simulink model "ADLK"  (R2022a)
settings: Solver=FixedStepDiscrete  StartTime=0.0  StopTime=10.0  FixedStep=0.01  RelTol=1e-3
libraries: DoorRatSts x4, ADLKDriver x2
settings Model: Creator=DELL  LastModifiedBy=DELL
settings DataIOCC: SaveFormat=StructureWithTime
settings OptimizationCC: DefaultParameterBehavior=Inlined  EnhancedBackFolding=on  PassReuseOutputArgsAs=Individual arguments  ZeroExternalMemoryAtStartup=off  ZeroInternalMemoryAtStartup=off  OptimizeBlockOrder=speed  DifferentSizesBufferReuse=on  OptimizationCustomize=off  EfficientTunableParamExpr=on
settings DebuggingCC: ParameterTunabilityLossMsg=error
settings ModelReferenceCC: ModelReferenceNumInstancesAllowed=Single
settings SFSimCC: MATLABDynamicMemAlloc=off
settings RTWCC: Description=AUTOSAR  SystemTargetFile=autosar.tlc  GenCodeOnly=on  TemplateMakefile=ert_default_tmf
settings CodeAppCC: ForceParamTrailComments=on  IgnoreCustomStorageClasses=off  OperatorAnnotations=on  SimulinkDataObjDesc=on  SFDataObjDesc=on  InsertBlockDesc=on
settings STFCustomTargetCC: TargetLangStandard=C99 (ISO)  MultiwordLength=256  ParMdlRefBuildCompliant=on  CompOptLevelCompliant=on  IncludeMdlTerminateFcn=off  CombineOutputUpdateFcns=on  SuppressErrorStatus=on  ERTCustomFileBanners=on  SupportNonFinite=off  SupportComplex=off  SupportContinuousTime=off  SupportNonInlinedSFcns=off  RemoveResetFunc=on  MATLABClassNameForMDSCustomization=Simulink.SoftwareTarget.ERTCustomization  AutosarCompliant=on  GRTInterface=off  UseToolchainInfoCompliant=on  LookupTableObjectStructAxisOrder=2,1,3,4,...  LUTObjectStructOrderEvenSpacing=Size,Table,Breakpoints  SystemTargetFile=autosar.tlc
settings ERTTargetCC: TargetLangStandard=C99 (ISO)  ConcurrentExecutionCompliant=off  IncludeMdlTerminateFcn=off  SuppressErrorStatus=on  SupportNonFinite=off  SupportComplex=off  ModelStepFunctionPrototypeControlCompliant=off  CPPClassGenCompliant=off  AutosarCompliant=on  LookupTableObjectStructAxisOrder=2,1,3,4,...  LUTObjectStructOrderEvenSpacing=Size,Table,Breakpoints  InlinedParameterPlacement=NonHierarchical  ERTCustomFileTemplate=example_file_process.tlc

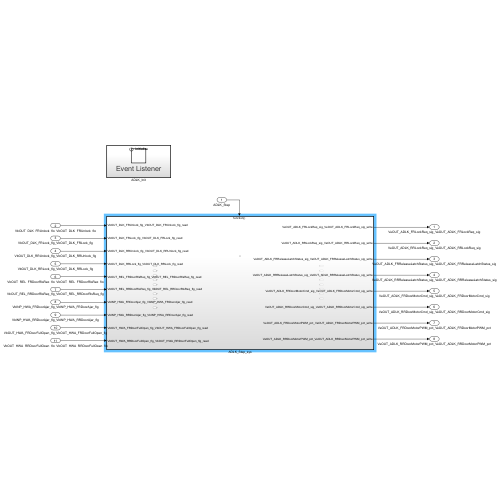
[thumbnail: Simulink's stored preview of the top-level diagram]
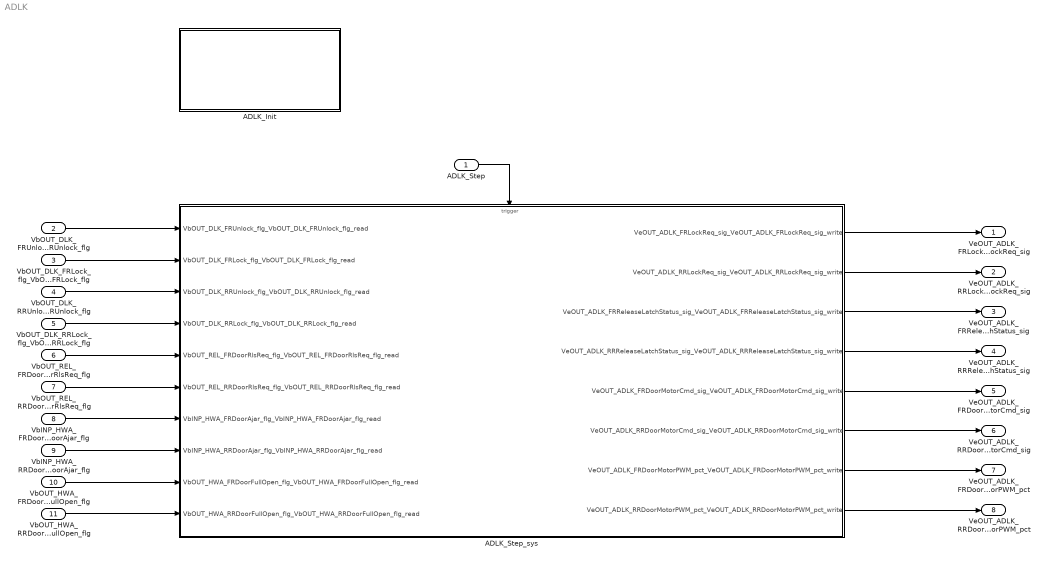
== system ADLK ==
  ADLK_Step : Inport  SampleTime=0.01  OutputFunctionCall=on
  VbOUT_DLK_FRUnlock_flg_VbOUT_DLK_FRUnlock_flg : Inport  Port=2  OutDataTypeStr=Boolean  PortDimensions=1
  VbOUT_DLK_FRLock_flg_VbOUT_DLK_FRLock_flg : Inport  Port=3  OutDataTypeStr=Boolean  PortDimensions=1
  VbOUT_DLK_RRUnlock_flg_VbOUT_DLK_RRUnlock_flg : Inport  Port=4  OutDataTypeStr=Boolean  PortDimensions=1
  VbOUT_DLK_RRLock_flg_VbOUT_DLK_RRLock_flg : Inport  Port=5  OutDataTypeStr=Boolean  PortDimensions=1
  VbOUT_REL_FRDoorRlsReq_flg_VbOUT_REL_FRDoorRlsReq_flg : Inport  Port=6  OutDataTypeStr=Boolean  PortDimensions=1
  VbOUT_REL_RRDoorRlsReq_flg_VbOUT_REL_RRDoorRlsReq_flg : Inport  Port=7  OutDataTypeStr=Boolean  PortDimensions=1
  VbINP_HWA_FRDoorAjar_flg_VbINP_HWA_FRDoorAjar_flg : Inport  Port=8  OutDataTypeStr=Boolean  PortDimensions=1
  VbINP_HWA_RRDoorAjar_flg_VbINP_HWA_RRDoorAjar_flg : Inport  Port=9  OutDataTypeStr=Boolean  PortDimensions=1
  VbOUT_HWA_FRDoorFullOpen_flg_VbOUT_HWA_FRDoorFullOpen_flg : Inport  Port=10  OutDataTypeStr=Boolean  PortDimensions=1
  VbOUT_HWA_RRDoorFullOpen_flg_VbOUT_HWA_RRDoorFullOpen_flg : Inport  Port=11  OutDataTypeStr=Boolean  PortDimensions=1
  ADLK_Init : Subsystem
  ADLK_Step_sys : Subsystem
  VeOUT_ADLK_FRLockReq_sig_VeOUT_ADLK_FRLockReq_sig : Outport  OutDataTypeStr=UInt8  PortDimensions=1
  VeOUT_ADLK_RRLockReq_sig_VeOUT_ADLK_RRLockReq_sig : Outport  Port=2  OutDataTypeStr=UInt8  PortDimensions=1
  VeOUT_ADLK_FRReleaseLatchStatus_sig_VeOUT_ADLK_FRReleaseLatchStatus_sig : Outport  Port=3  OutDataTypeStr=UInt8  PortDimensions=1
  VeOUT_ADLK_RRReleaseLatchStatus_sig_VeOUT_ADLK_RRReleaseLatchStatus_sig : Outport  Port=4  OutDataTypeStr=UInt8  PortDimensions=1
  VeOUT_ADLK_FRDoorMotorCmd_sig_VeOUT_ADLK_FRDoorMotorCmd_sig : Outport  Port=5  OutDataTypeStr=UInt8  PortDimensions=1
  VeOUT_ADLK_RRDoorMotorCmd_sig_VeOUT_ADLK_RRDoorMotorCmd_sig : Outport  Port=6  OutDataTypeStr=UInt8  PortDimensions=1
  VeOUT_ADLK_FRDoorMotorPWM_pct_VeOUT_ADLK_FRDoorMotorPWM_pct : Outport  Port=7  OutDataTypeStr=UInt8  PortDimensions=1
  VeOUT_ADLK_RRDoorMotorPWM_pct_VeOUT_ADLK_RRDoorMotorPWM_pct : Outport  Port=8  OutDataTypeStr=UInt8  PortDimensions=1
  wires:
  VbOUT_DLK_FRUnlock_flg_VbOUT_DLK_FRUnlock_flg/1 -> ADLK_Step_sys/1(VbOUT_DLK_FRUnlock_flg_VbOUT_DLK_FRUnlock_flg_read)
  VbOUT_DLK_FRLock_flg_VbOUT_DLK_FRLock_flg/1 -> ADLK_Step_sys/2(VbOUT_DLK_FRLock_flg_VbOUT_DLK_FRLock_flg_read)
  VbOUT_DLK_RRUnlock_flg_VbOUT_DLK_RRUnlock_flg/1 -> ADLK_Step_sys/3(VbOUT_DLK_RRUnlock_flg_VbOUT_DLK_RRUnlock_flg_read)
  VbOUT_DLK_RRLock_flg_VbOUT_DLK_RRLock_flg/1 -> ADLK_Step_sys/4(VbOUT_DLK_RRLock_flg_VbOUT_DLK_RRLock_flg_read)
  VbOUT_REL_FRDoorRlsReq_flg_VbOUT_REL_FRDoorRlsReq_flg/1 -> ADLK_Step_sys/5(VbOUT_REL_FRDoorRlsReq_flg_VbOUT_REL_FRDoorRlsReq_flg_read)
  VbOUT_REL_RRDoorRlsReq_flg_VbOUT_REL_RRDoorRlsReq_flg/1 -> ADLK_Step_sys/6(VbOUT_REL_RRDoorRlsReq_flg_VbOUT_REL_RRDoorRlsReq_flg_read)
  VbINP_HWA_FRDoorAjar_flg_VbINP_HWA_FRDoorAjar_flg/1 -> ADLK_Step_sys/7(VbINP_HWA_FRDoorAjar_flg_VbINP_HWA_FRDoorAjar_flg_read)
  VbINP_HWA_RRDoorAjar_flg_VbINP_HWA_RRDoorAjar_flg/1 -> ADLK_Step_sys/8(VbINP_HWA_RRDoorAjar_flg_VbINP_HWA_RRDoorAjar_flg_read)
  VbOUT_HWA_FRDoorFullOpen_flg_VbOUT_HWA_FRDoorFullOpen_flg/1 -> ADLK_Step_sys/9(VbOUT_HWA_FRDoorFullOpen_flg_VbOUT_HWA_FRDoorFullOpen_flg_read)
  VbOUT_HWA_RRDoorFullOpen_flg_VbOUT_HWA_RRDoorFullOpen_flg/1 -> ADLK_Step_sys/10(VbOUT_HWA_RRDoorFullOpen_flg_VbOUT_HWA_RRDoorFullOpen_flg_read)
  ADLK_Step_sys/1(VeOUT_ADLK_FRLockReq_sig_VeOUT_ADLK_FRLockReq_sig_write) -> VeOUT_ADLK_FRLockReq_sig_VeOUT_ADLK_FRLockReq_sig/1
  ADLK_Step_sys/2(VeOUT_ADLK_RRLockReq_sig_VeOUT_ADLK_RRLockReq_sig_write) -> VeOUT_ADLK_RRLockReq_sig_VeOUT_ADLK_RRLockReq_sig/1
  ADLK_Step_sys/3(VeOUT_ADLK_FRReleaseLatchStatus_sig_VeOUT_ADLK_FRReleaseLatchStatus_sig_write) -> VeOUT_ADLK_FRReleaseLatchStatus_sig_VeOUT_ADLK_FRReleaseLatchStatus_sig/1
  ADLK_Step_sys/4(VeOUT_ADLK_RRReleaseLatchStatus_sig_VeOUT_ADLK_RRReleaseLatchStatus_sig_write) -> VeOUT_ADLK_RRReleaseLatchStatus_sig_VeOUT_ADLK_RRReleaseLatchStatus_sig/1
  ADLK_Step_sys/5(VeOUT_ADLK_FRDoorMotorCmd_sig_VeOUT_ADLK_FRDoorMotorCmd_sig_write) -> VeOUT_ADLK_FRDoorMotorCmd_sig_VeOUT_ADLK_FRDoorMotorCmd_sig/1
  ADLK_Step_sys/6(VeOUT_ADLK_RRDoorMotorCmd_sig_VeOUT_ADLK_RRDoorMotorCmd_sig_write) -> VeOUT_ADLK_RRDoorMotorCmd_sig_VeOUT_ADLK_RRDoorMotorCmd_sig/1
  ADLK_Step_sys/7(VeOUT_ADLK_FRDoorMotorPWM_pct_VeOUT_ADLK_FRDoorMotorPWM_pct_write) -> VeOUT_ADLK_FRDoorMotorPWM_pct_VeOUT_ADLK_FRDoorMotorPWM_pct/1
  ADLK_Step_sys/8(VeOUT_ADLK_RRDoorMotorPWM_pct_VeOUT_ADLK_RRDoorMotorPWM_pct_write) -> VeOUT_ADLK_RRDoorMotorPWM_pct_VeOUT_ADLK_RRDoorMotorPWM_pct/1
  ADLK_Step/1 -> ADLK_Step_sys/Trigger

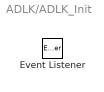
== system ADLK/ADLK_Init ==
  Event Listener : EventListener  EventName=reset

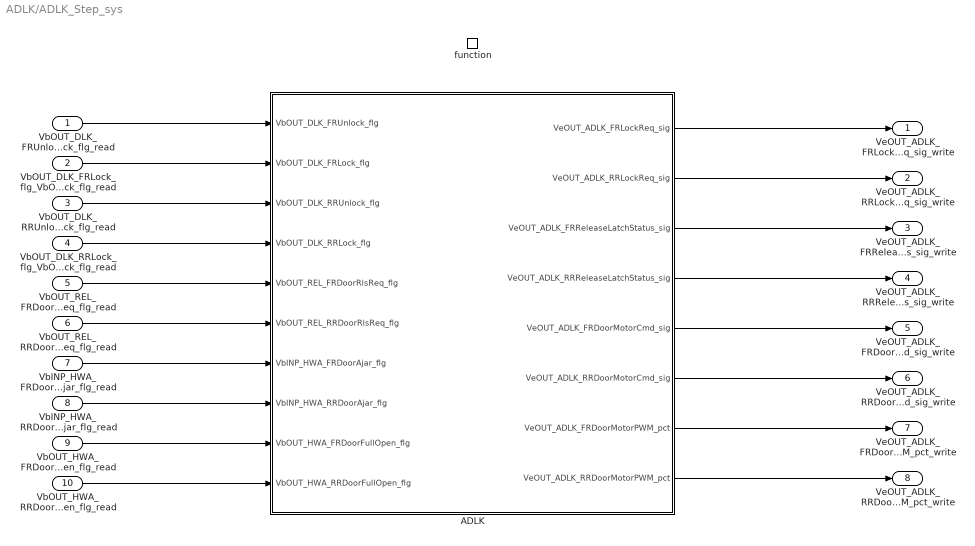
== system ADLK/ADLK_Step_sys ==
  VbOUT_DLK_FRUnlock_flg_VbOUT_DLK_FRUnlock_flg_read : Inport
  VbOUT_DLK_FRLock_flg_VbOUT_DLK_FRLock_flg_read : Inport  Port=2
  VbOUT_DLK_RRUnlock_flg_VbOUT_DLK_RRUnlock_flg_read : Inport  Port=3
  VbOUT_DLK_RRLock_flg_VbOUT_DLK_RRLock_flg_read : Inport  Port=4
  VbOUT_REL_FRDoorRlsReq_flg_VbOUT_REL_FRDoorRlsReq_flg_read : Inport  Port=5
  VbOUT_REL_RRDoorRlsReq_flg_VbOUT_REL_RRDoorRlsReq_flg_read : Inport  Port=6
  VbINP_HWA_FRDoorAjar_flg_VbINP_HWA_FRDoorAjar_flg_read : Inport  Port=7
  VbINP_HWA_RRDoorAjar_flg_VbINP_HWA_RRDoorAjar_flg_read : Inport  Port=8
  VbOUT_HWA_FRDoorFullOpen_flg_VbOUT_HWA_FRDoorFullOpen_flg_read : Inport  Port=9
  VbOUT_HWA_RRDoorFullOpen_flg_VbOUT_HWA_RRDoorFullOpen_flg_read : Inport  Port=10
  function : TriggerPort  TriggerType=function-call  VariantControl=(inherit)  SampleTimeType=periodic  SampleTime=-1
  ADLK : Subsystem
  VeOUT_ADLK_FRLockReq_sig_VeOUT_ADLK_FRLockReq_sig_write : Outport
      settings: EnsureOutportIsVirtual=on
  VeOUT_ADLK_RRLockReq_sig_VeOUT_ADLK_RRLockReq_sig_write : Outport  Port=2
      settings: EnsureOutportIsVirtual=on
  VeOUT_ADLK_FRReleaseLatchStatus_sig_VeOUT_ADLK_FRReleaseLatchStatus_sig_write : Outport  Port=3
      settings: EnsureOutportIsVirtual=on
  VeOUT_ADLK_RRReleaseLatchStatus_sig_VeOUT_ADLK_RRReleaseLatchStatus_sig_write : Outport  Port=4
      settings: EnsureOutportIsVirtual=on
  VeOUT_ADLK_FRDoorMotorCmd_sig_VeOUT_ADLK_FRDoorMotorCmd_sig_write : Outport  Port=5
      settings: EnsureOutportIsVirtual=on
  VeOUT_ADLK_RRDoorMotorCmd_sig_VeOUT_ADLK_RRDoorMotorCmd_sig_write : Outport  Port=6
      settings: EnsureOutportIsVirtual=on
  VeOUT_ADLK_FRDoorMotorPWM_pct_VeOUT_ADLK_FRDoorMotorPWM_pct_write : Outport  Port=7
      settings: EnsureOutportIsVirtual=on
  VeOUT_ADLK_RRDoorMotorPWM_pct_VeOUT_ADLK_RRDoorMotorPWM_pct_write : Outport  Port=8
      settings: EnsureOutportIsVirtual=on
  wires:
  VbOUT_DLK_FRUnlock_flg_VbOUT_DLK_FRUnlock_flg_read/1 -> ADLK/1(VbOUT_DLK_FRUnlock_flg)
  VbOUT_DLK_FRLock_flg_VbOUT_DLK_FRLock_flg_read/1 -> ADLK/2(VbOUT_DLK_FRLock_flg)
  VbOUT_DLK_RRUnlock_flg_VbOUT_DLK_RRUnlock_flg_read/1 -> ADLK/3(VbOUT_DLK_RRUnlock_flg)
  VbOUT_DLK_RRLock_flg_VbOUT_DLK_RRLock_flg_read/1 -> ADLK/4(VbOUT_DLK_RRLock_flg)
  VbOUT_REL_FRDoorRlsReq_flg_VbOUT_REL_FRDoorRlsReq_flg_read/1 -> ADLK/5(VbOUT_REL_FRDoorRlsReq_flg)
  VbOUT_REL_RRDoorRlsReq_flg_VbOUT_REL_RRDoorRlsReq_flg_read/1 -> ADLK/6(VbOUT_REL_RRDoorRlsReq_flg)
  VbINP_HWA_FRDoorAjar_flg_VbINP_HWA_FRDoorAjar_flg_read/1 -> ADLK/7(VbINP_HWA_FRDoorAjar_flg)
  VbINP_HWA_RRDoorAjar_flg_VbINP_HWA_RRDoorAjar_flg_read/1 -> ADLK/8(VbINP_HWA_RRDoorAjar_flg)
  VbOUT_HWA_FRDoorFullOpen_flg_VbOUT_HWA_FRDoorFullOpen_flg_read/1 -> ADLK/9(VbOUT_HWA_FRDoorFullOpen_flg)
  VbOUT_HWA_RRDoorFullOpen_flg_VbOUT_HWA_RRDoorFullOpen_flg_read/1 -> ADLK/10(VbOUT_HWA_RRDoorFullOpen_flg)
  ADLK/1(VeOUT_ADLK_FRLockReq_sig) -> VeOUT_ADLK_FRLockReq_sig_VeOUT_ADLK_FRLockReq_sig_write/1
  ADLK/2(VeOUT_ADLK_RRLockReq_sig) -> VeOUT_ADLK_RRLockReq_sig_VeOUT_ADLK_RRLockReq_sig_write/1
  ADLK/3(VeOUT_ADLK_FRReleaseLatchStatus_sig) -> VeOUT_ADLK_FRReleaseLatchStatus_sig_VeOUT_ADLK_FRReleaseLatchStatus_sig_write/1
  ADLK/4(VeOUT_ADLK_RRReleaseLatchStatus_sig) -> VeOUT_ADLK_RRReleaseLatchStatus_sig_VeOUT_ADLK_RRReleaseLatchStatus_sig_write/1
  ADLK/5(VeOUT_ADLK_FRDoorMotorCmd_sig) -> VeOUT_ADLK_FRDoorMotorCmd_sig_VeOUT_ADLK_FRDoorMotorCmd_sig_write/1
  ADLK/6(VeOUT_ADLK_RRDoorMotorCmd_sig) -> VeOUT_ADLK_RRDoorMotorCmd_sig_VeOUT_ADLK_RRDoorMotorCmd_sig_write/1
  ADLK/7(VeOUT_ADLK_FRDoorMotorPWM_pct) -> VeOUT_ADLK_FRDoorMotorPWM_pct_VeOUT_ADLK_FRDoorMotorPWM_pct_write/1
  ADLK/8(VeOUT_ADLK_RRDoorMotorPWM_pct) -> VeOUT_ADLK_RRDoorMotorPWM_pct_VeOUT_ADLK_RRDoorMotorPWM_pct_write/1

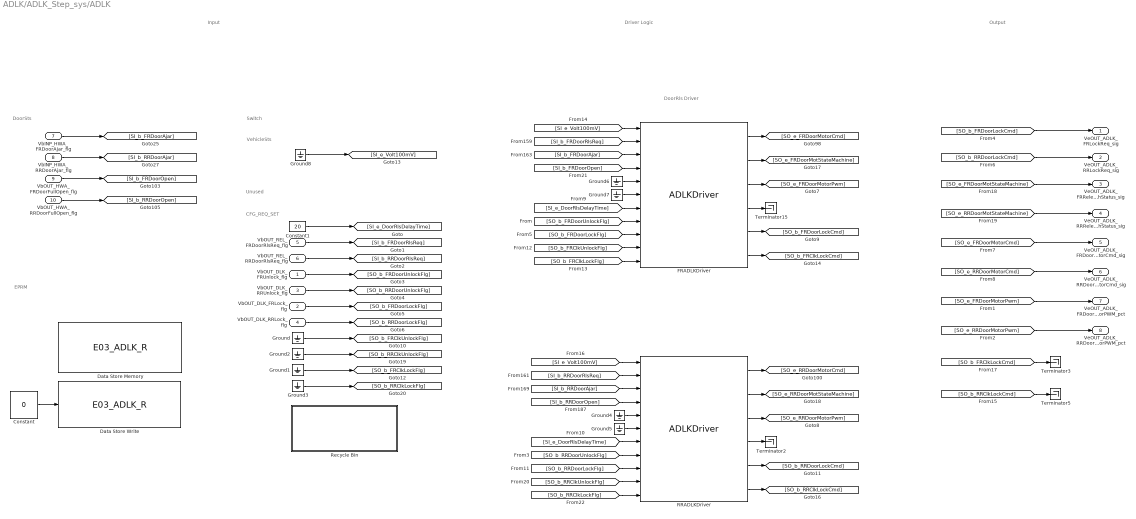
== system ADLK/ADLK_Step_sys/ADLK ==
  note: VehicleSts
  note: Input
  note: Output
  note: EPRM
  note: Driver Logic
  note: DoorRls Driver
  note: Switch
  note: DoorSts
  note: CFG_REQ_SET
  note: Unused
  VbOUT_DLK_FRUnlock_flg : Inport
  VbOUT_DLK_FRLock_flg : Inport  Port=2
  VbOUT_DLK_RRUnlock_flg : Inport  Port=3
  VbOUT_DLK_RRLock_flg : Inport  Port=4
  VbOUT_REL_FRDoorRlsReq_flg : Inport  Port=5
  VbOUT_REL_RRDoorRlsReq_flg : Inport  Port=6
  VbINP_HWA_FRDoorAjar_flg : Inport  Port=7
  VbINP_HWA_RRDoorAjar_flg : Inport  Port=8
  VbOUT_HWA_FRDoorFullOpen_flg : Inport  Port=9
  VbOUT_HWA_RRDoorFullOpen_flg : Inport  Port=10
  Constant : Constant  Value=0  OutDataTypeStr=uint8
  Constant1 : Constant  Value=20  OutDataTypeStr=uint8
  Data Store Memory : DataStoreMemory  DataStoreName=E03_ADLK_R  WriteAfterWriteMsg=warning  ShowAdditionalParam=off  OutDataTypeStr=uint8
  Data Store Write : DataStoreWrite  DataStoreName=E03_ADLK_R  IndexOptions=Index vector (dialog)  Indices=1  OutputSizes=1
  FRADLKDriver : ADLKDriver/ADLKDriver  SystemSampleTime=-1  VariantActivationTime=update diagram  Latency=0  AutoFrameSizeCalculation=off
  Ground{,1..8} (9 alike) : Ground
  RRADLKDriver : ADLKDriver/ADLKDriver  SystemSampleTime=-1  VariantActivationTime=update diagram  Latency=0  AutoFrameSizeCalculation=off
  Recycle Bin : Subsystem
  Terminator{2..3,5,15} (4 alike) : Terminator
  VeOUT_ADLK_FRLockReq_sig : Outport
  VeOUT_ADLK_RRLockReq_sig : Outport  Port=2
  VeOUT_ADLK_FRReleaseLatchStatus_sig : Outport  Port=3
  VeOUT_ADLK_RRReleaseLatchStatus_sig : Outport  Port=4
  VeOUT_ADLK_FRDoorMotorCmd_sig : Outport  Port=5
  VeOUT_ADLK_RRDoorMotorCmd_sig : Outport  Port=6
  VeOUT_ADLK_FRDoorMotorPWM_pct : Outport  Port=7
  VeOUT_ADLK_RRDoorMotorPWM_pct : Outport  Port=8
  wires:
  Constant/1 -> Data Store Write/1
  [SI_b_RRDoorOpen] -> RRADLKDriver/4
  [SI_b_RRDoorAjar] -> RRADLKDriver/3
  [SI_b_RRDoorRlsReq] -> RRADLKDriver/2
  [SI_e_Volt100mV] -> RRADLKDriver/1
  [SI_b_FRDoorAjar] -> FRADLKDriver/3
  [SI_b_FRDoorRlsReq] -> FRADLKDriver/2
  [SI_b_FRDoorOpen] -> FRADLKDriver/4
  [SI_e_DoorRlsDelayTime] -> FRADLKDriver/7
  Ground4/1 -> RRADLKDriver/5
  Ground5/1 -> RRADLKDriver/6
  Ground6/1 -> FRADLKDriver/5
  Ground7/1 -> FRADLKDriver/6
  [SI_e_Volt100mV] -> FRADLKDriver/1
  Constant1/1 -> [SI_e_DoorRlsDelayTime]
  [SI_e_DoorRlsDelayTime] -> RRADLKDriver/7
  [SO_b_FRDoorLockFlg] -> FRADLKDriver/9
  [SO_b_FRDoorUnlockFlg] -> FRADLKDriver/8
  [SO_b_RRDoorUnlockFlg] -> RRADLKDriver/8
  [SO_b_RRDoorLockFlg] -> RRADLKDriver/9
  [SO_b_FRClkUnlockFlg] -> FRADLKDriver/10
  [SO_b_FRClkLockFlg] -> FRADLKDriver/11
  Ground/1 -> [SO_b_FRClkUnlockFlg]
  Ground1/1 -> [SO_b_FRClkLockFlg]
  [SO_b_FRDoorLockCmd] -> VeOUT_ADLK_FRLockReq_sig/1
  [SO_b_RRDoorLockCmd] -> VeOUT_ADLK_RRLockReq_sig/1
  [SO_e_FRDoorMotStateMachine] -> VeOUT_ADLK_FRReleaseLatchStatus_sig/1
  [SO_e_RRDoorMotStateMachine] -> VeOUT_ADLK_RRReleaseLatchStatus_sig/1
  [SO_b_FRClkLockCmd] -> Terminator3/1
  [SO_b_RRClkLockCmd] -> Terminator5/1
  Ground2/1 -> [SO_b_RRClkUnlockFlg]
  Ground3/1 -> [SO_b_RRClkLockFlg]
  [SO_b_RRClkUnlockFlg] -> RRADLKDriver/10
  [SO_b_RRClkLockFlg] -> RRADLKDriver/11
  VbINP_HWA_FRDoorAjar_flg/1 -> [SI_b_FRDoorAjar]
  VbINP_HWA_RRDoorAjar_flg/1 -> [SI_b_RRDoorAjar]
  VbOUT_HWA_FRDoorFullOpen_flg/1 -> [SI_b_FRDoorOpen]
  VbOUT_HWA_RRDoorFullOpen_flg/1 -> [SI_b_RRDoorOpen]
  VbOUT_REL_FRDoorRlsReq_flg/1 -> [SI_b_FRDoorRlsReq]
  VbOUT_REL_RRDoorRlsReq_flg/1 -> [SI_b_RRDoorRlsReq]
  VbOUT_DLK_FRUnlock_flg/1 -> [SO_b_FRDoorUnlockFlg]
  VbOUT_DLK_RRUnlock_flg/1 -> [SO_b_RRDoorUnlockFlg]
  VbOUT_DLK_FRLock_flg/1 -> [SO_b_FRDoorLockFlg]
  VbOUT_DLK_RRLock_flg/1 -> [SO_b_RRDoorLockFlg]
  RRADLKDriver/3 -> [SO_e_RRDoorMotorPwm]
  [SO_e_FRDoorMotorCmd] -> VeOUT_ADLK_FRDoorMotorCmd_sig/1
  [SO_e_RRDoorMotorCmd] -> VeOUT_ADLK_RRDoorMotorCmd_sig/1
  [SO_e_FRDoorMotorPwm] -> VeOUT_ADLK_FRDoorMotorPWM_pct/1
  [SO_e_RRDoorMotorPwm] -> VeOUT_ADLK_RRDoorMotorPWM_pct/1
  FRADLKDriver/3 -> [SO_e_FRDoorMotorPwm]
  FRADLKDriver/1 -> [SO_e_FRDoorMotorCmd]
  FRADLKDriver/4 -> Terminator15/1
  FRADLKDriver/6 -> [SO_b_FRClkLockCmd]
  FRADLKDriver/5 -> [SO_b_FRDoorLockCmd]
  FRADLKDriver/2 -> [SO_e_FRDoorMotStateMachine]
  RRADLKDriver/1 -> [SO_e_RRDoorMotorCmd]
  RRADLKDriver/6 -> [SO_b_RRClkLockCmd]
  RRADLKDriver/5 -> [SO_b_RRDoorLockCmd]
  RRADLKDriver/2 -> [SO_e_RRDoorMotStateMachine]
  RRADLKDriver/4 -> Terminator2/1
  Ground8/1 -> [SI_e_Volt100mV]

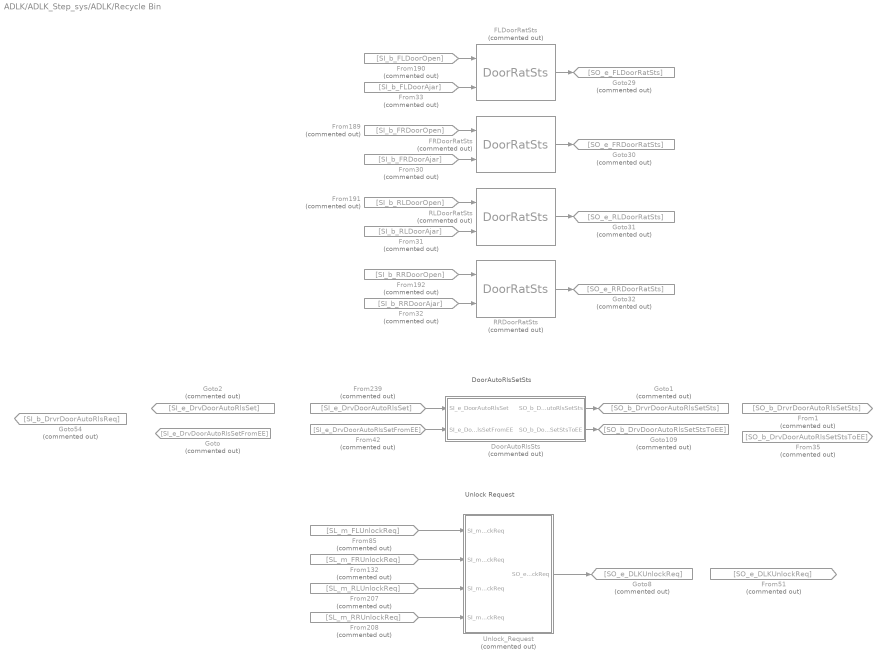
== system ADLK/ADLK_Step_sys/ADLK/Recycle Bin ==
  note: DoorAutoRlsSetSts
  note: Unlock Request
  DoorAutoRlsSts : Stateflow chart  Commented=on  TreatAsAtomicUnit=on
  FLDoorRatSts : DoorRatSts/DoorRatSts  Commented=on  SystemSampleTime=-1  VariantActivationTime=update diagram  Latency=0  AutoFrameSizeCalculation=off
  FRDoorRatSts : DoorRatSts/DoorRatSts  Commented=on  SystemSampleTime=-1  VariantActivationTime=update diagram  Latency=0  AutoFrameSizeCalculation=off
  From1 : From  Commented=on  GotoTag=SO_b_DrvrDoorAutoRlsSetSts
  From132 : From  Commented=on  GotoTag=SL_m_FRUnlockReq
  From189 : From  Commented=on  GotoTag=SI_b_FRDoorOpen
  From190 : From  Commented=on  GotoTag=SI_b_FLDoorOpen
  From191 : From  Commented=on  GotoTag=SI_b_RLDoorOpen
  From192 : From  Commented=on  GotoTag=SI_b_RRDoorOpen
  From207 : From  Commented=on  GotoTag=SL_m_RLUnlockReq
  From208 : From  Commented=on  GotoTag=SL_m_RRUnlockReq
  From239 : From  Commented=on  GotoTag=SI_e_DrvDoorAutoRlsSet
  From30 : From  Commented=on  GotoTag=SI_b_FRDoorAjar
  From31 : From  Commented=on  GotoTag=SI_b_RLDoorAjar
  From32 : From  Commented=on  GotoTag=SI_b_RRDoorAjar
  From33 : From  Commented=on  GotoTag=SI_b_FLDoorAjar
  From35 : From  Commented=on  GotoTag=SO_b_DrvDoorAutoRlsSetStsToEE
  From42 : From  Commented=on  GotoTag=SI_e_DrvDoorAutoRlsSetFromEE
  From51 : From  Commented=on  GotoTag=SO_e_DLKUnlockReq
  From85 : From  Commented=on  GotoTag=SL_m_FLUnlockReq
  Goto : Goto  Commented=on  GotoTag=SI_e_DrvDoorAutoRlsSetFromEE
  Goto1 : Goto  Commented=on  GotoTag=SO_b_DrvrDoorAutoRlsSetSts
  Goto109 : Goto  Commented=on  GotoTag=SO_b_DrvDoorAutoRlsSetStsToEE
  Goto2 : Goto  Commented=on  GotoTag=SI_e_DrvDoorAutoRlsSet
  Goto29 : Goto  Commented=on  GotoTag=SO_e_FLDoorRatSts
  Goto30 : Goto  Commented=on  GotoTag=SO_e_FRDoorRatSts
  Goto31 : Goto  Commented=on  GotoTag=SO_e_RLDoorRatSts
  Goto32 : Goto  Commented=on  GotoTag=SO_e_RRDoorRatSts
  Goto54 : Goto  Commented=on  GotoTag=SI_b_DrvrDoorAutoRlsReq
  Goto8 : Goto  Commented=on  GotoTag=SO_e_DLKUnlockReq
  RLDoorRatSts : DoorRatSts/DoorRatSts  Commented=on  SystemSampleTime=-1  VariantActivationTime=update diagram  Latency=0  AutoFrameSizeCalculation=off
  RRDoorRatSts : DoorRatSts/DoorRatSts  Commented=on  SystemSampleTime=-1  VariantActivationTime=update diagram  Latency=0  AutoFrameSizeCalculation=off
  Unlock_Request : Stateflow chart  Commented=on  TreatAsAtomicUnit=on
  wires:
  FLDoorRatSts/1 -> Goto29/1
  From191/1 -> RLDoorRatSts/1
  FRDoorRatSts/1 -> Goto30/1
  From190/1 -> FLDoorRatSts/1
  From192/1 -> RRDoorRatSts/1
  From189/1 -> FRDoorRatSts/1
  RRDoorRatSts/1 -> Goto32/1
  RLDoorRatSts/1 -> Goto31/1
  From30/1 -> FRDoorRatSts/2
  From32/1 -> RRDoorRatSts/2
  From31/1 -> RLDoorRatSts/2
  From33/1 -> FLDoorRatSts/2
  DoorAutoRlsSts/1(SO_b_DoorAutoRlsSetSts) -> Goto1/1
  DoorAutoRlsSts/2(SO_b_DoorAutoRlsSetStsToEE) -> Goto109/1
  From42/1 -> DoorAutoRlsSts/2(SI_e_DoorAutoRlsSetFromEE)
  From239/1 -> DoorAutoRlsSts/1(SI_e_DoorAutoRlsSet)
  From132/1 -> Unlock_Request/2(SI_m_FRUnlockReq)
  From208/1 -> Unlock_Request/4(SI_m_RRUnlockReq)
  From207/1 -> Unlock_Request/3(SI_m_RLUnlockReq)
  Unlock_Request/1(SO_e_UnlockReq) -> Goto8/1
  From85/1 -> Unlock_Request/1(SI_m_FLUnlockReq)

== stateflow chart ADLK/ADLK_Step_sys/ADLK/Recycle Bin/DoorAutoRlsSts ==
  state DoorLockSet
    (default) -> (junction 127) : /* DoorLockSet */
    DoorLockSet -> (junction 127)
    (junction 127) -> (junction 128) [order 1] : [SI_e_DoorAutoRlsSet == 1 || ...
        | (SI_e_DoorAutoRlsSet != 2 && SL_e_DoorAutoRlsSetBackup == 1)]
    (junction 127) -> (junction 129) [order 2]
    (junction 128) -> (junction 136) : {SO_b_DoorAutoRlsSetSts = 1; ...
        | SO_b_DoorAutoRlsSetStsToEE = 1; ...
        | SL_e_DoorAutoRlsSetBackup = 1}
    (junction 129) -> (junction 130) [order 1] : [SI_e_DoorAutoRlsSet == 2 || ...
        | (SI_e_DoorAutoRlsSet != 1 && SL_e_DoorAutoRlsSetBackup == 2)]
    (junction 129) -> (junction 131) [order 2]
    (junction 130) -> (junction 135) : {SO_b_DoorAutoRlsSetSts = 0; ...
        | SO_b_DoorAutoRlsSetStsToEE = 0; ...
        | SL_e_DoorAutoRlsSetBackup = 2}
    (junction 131) -> (junction 132) [order 1] : [SI_e_DoorAutoRlsSetFromEE == 1]
    (junction 131) -> (junction 151) [order 2]
    (junction 132) -> (junction 134) : {SO_b_DoorAutoRlsSetSts = 1; ...
        | SO_b_DoorAutoRlsSetStsToEE = 1;}
    (junction 151) -> (junction 159) [order 1] : [SI_e_DoorAutoRlsSetFromEE == 0]
    (junction 151) -> (junction 133) [order 2]
    (junction 159) -> (junction 160) : {SO_b_DoorAutoRlsSetSts = 0; ...
        | SO_b_DoorAutoRlsSetStsToEE = 0;}
    (junction 160) -> (junction 133)
    (junction 134) -> (junction 160)
    (junction 135) -> (junction 134)
    (junction 136) -> (junction 135)
    (junction 133) -> (junction 137)
  data: SO_b_DoorAutoRlsSetSts output boolean; SI_e_DoorAutoRlsSet input uint8; SI_e_DoorAutoRlsSetFromEE input uint8; SO_b_DoorAutoRlsSetStsToEE output boolean; SL_e_DoorAutoRlsSetBackup local uint8 =0

== stateflow chart ADLK/ADLK_Step_sys/ADLK/Recycle Bin/Unlock_Request ==
  state req = GetDrvUnlockReq [function]
    (default) -> (junction 216)
    (junction 216) -> (junction 217) [order 1] : [SI_m_FLUnlockReq == Unlock_PE]
    (junction 216) -> (junction 218) [order 2]
    (junction 217) -> (junction 222) : {req = Unlock_PE;}
    (junction 218) -> (junction 219) [order 1] : [SI_m_FLUnlockReq == Unlock_Req]
    (junction 218) -> (junction 220) [order 2] : {req = Unlock_Idle;}
    (junction 219) -> (junction 221) : {req = Unlock_Req;}
    (junction 221) -> (junction 220)
    (junction 222) -> (junction 221)
    (junction 220) -> (junction 223)
  state UnlockReq
    (default) -> (junction 185)
    UnlockReq -> (junction 185)
    (junction 185) -> (junction 186) [order 1] : [(GetDrvUnlockReq() == Unlock_Req && GetPassUnlockReq() == Unlock_Req) || ...
        | GetDrvUnlockReq() == Unlock_PE || ...
        | GetPassUnlockReq() == Unlock_PE]
    (junction 185) -> (junction 187) [order 2]
    (junction 186) -> (junction 194) : {SO_e_UnlockReq = 3;}
    (junction 187) -> (junction 188) [order 1] : [GetDrvUnlockReq() == Unlock_Idle && ...
        | GetPassUnlockReq() == Unlock_Req]
    (junction 187) -> (junction 189) [order 2]
    (junction 188) -> (junction 193) : {SO_e_UnlockReq = 2;}
    (junction 189) -> (junction 190) [order 1] : [GetDrvUnlockReq() == Unlock_Req && ...
        | GetPassUnlockReq() == Unlock_Idle]
    (junction 189) -> (junction 191) [order 2] : {SO_e_UnlockReq = 0;}
    (junction 190) -> (junction 192) : {SO_e_UnlockReq = 1;}
    (junction 192) -> (junction 191)
    (junction 193) -> (junction 192)
    (junction 194) -> (junction 193)
    (junction 191) -> (junction 195)
  state req = GetPassUnlockReq [function]
    (default) -> (junction 232)
    (junction 232) -> (junction 228) [order 1] : [SI_m_FRUnlockReq == Unlock_PE || ...
        | SI_m_RLUnlockReq == Unlock_PE || ...
        | SI_m_RRUnlockReq == Unlock_PE]
    (junction 232) -> (junction 234) [order 2]
    (junction 228) -> (junction 238) : {req = Unlock_PE;}
    (junction 234) -> (junction 237) [order 1] : [SI_m_FRUnlockReq == Unlock_Req || ...
        | SI_m_RLUnlockReq == Unlock_Req || ...
        | SI_m_RRUnlockReq == Unlock_Req]
    (junction 234) -> (junction 240) [order 2] : {req = Unlock_Idle;}
    (junction 237) -> (junction 241) : {req = Unlock_Req;}
    (junction 241) -> (junction 240)
    (junction 238) -> (junction 241)
    (junction 240) -> (junction 239)
  data: req function_output double; req function_output double; SO_e_UnlockReq output uint8; SI_m_FLUnlockReq input Enum: Unlock_Req_E; SI_m_FRUnlockReq input Enum: Unlock_Req_E; SI_m_RLUnlockReq input Enum: Unlock_Req_E; SI_m_RRUnlockReq input Enum: Unlock_Req_E
